simulink model "quadcopter_wind"  (Simulink 9.0)
settings: Solver=ode45  StartTime=0.0  StopTime=30  FixedStep=0.001  RelTol=1e-3  EnableMultiTasking=on
values from neighbouring files (symbols this model uses):
  C = 1    [control_params.m]
  f_phi = 10    [control_params.m]
  f_psi = 0.1    [control_params.m]
  f_theta = 0.1    [control_params.m]
  f_x = 10    [control_params.m]
  f_y = 10    [control_params.m]
  f_z = 10    [control_params.m]
  g = 9.8    [control_params.m]
  J_1 = 1    [control_params.m]
  J_2 = 1    [control_params.m]
  J_3 = 1    [control_params.m]
  l = 0.5    [control_params.m]
  m = 1    [control_params.m]
  mu_1 = 10    [control_params.m]
  mu_2 = 2    [control_params.m]
  mu_3 = 2    [control_params.m]
  mu_4 = 10    [control_params.m]
  mu_5 = 10    [control_params.m]
  mu_6 = 10    [control_params.m]
  phi_desired = 20    [control_params.m]
  sigma_1 = 30    [control_params.m]
  sigma_2 = 30    [control_params.m]
  sigma_3 = 30    [control_params.m]
  sigma_4 = 30    [control_params.m]
  sigma_5 = 30    [control_params.m]
  sigma_6 = 30    [control_params.m]
  x_desired = 10    [control_params.m]
  y_desired = 20    [control_params.m]
  z_desired = 30    [control_params.m]
settings Model: Creator=Oleg Borisov  LastModifiedBy=broth
settings DataIOCC: LimitDataPoints=on  SignalLoggingSaveFormat=ModelDataLogs
settings OptimizationCC: ExpressionDepthLimit=2147483647
settings DebuggingCC: SolverPrmCheckMsg=warning  FcnCallInpInsideContextMsg=warning  StateNameClashWarn=warning
settings GRTTargetCC: GeneratePreprocessorConditionals=Disable all  CombineOutputUpdateFcns=off  GRTInterface=on

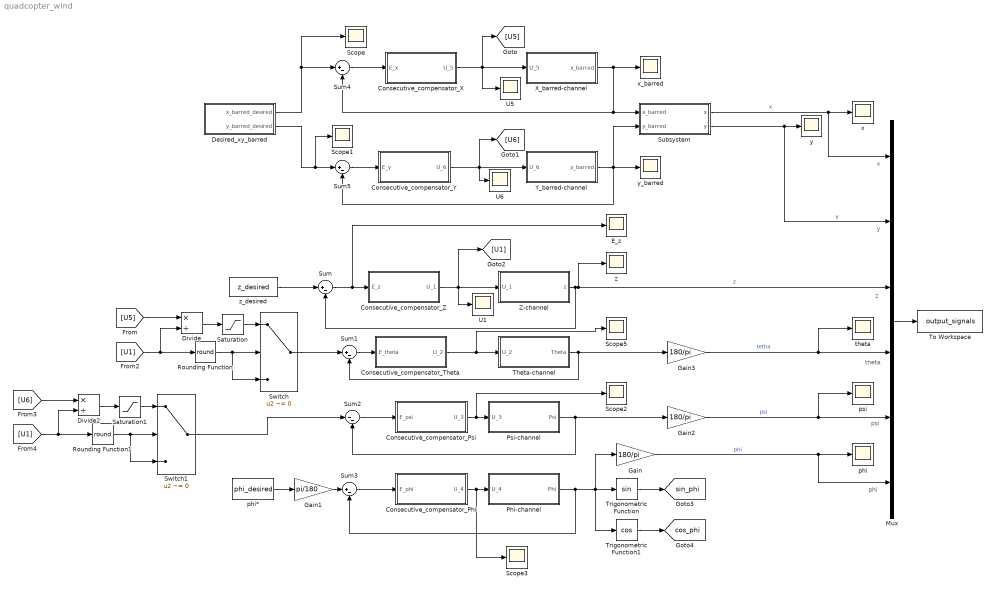
== system quadcopter_wind ==
  note: z
  note: y
  note: x
  note: theta
  note: psi
  note: phi
  Consecutive_compensator_Phi : Subsystem
  Consecutive_compensator_Psi : Subsystem
  Consecutive_compensator_Theta : Subsystem
  Consecutive_compensator_X : Subsystem
  Consecutive_compensator_Y : Subsystem
  Consecutive_compensator_Z : Subsystem
  Desired_xy_barred : Subsystem
  Divide : Product  Inputs=*/
  Divide2 : Product  Inputs=*/
  E_z : Scope
  Gain : Gain  Gain=180/pi
  Gain1 : Gain  Gain=pi/180
  Gain2 : Gain  Gain=180/pi
  Gain3 : Gain  Gain=180/pi
  Mux : Mux  Inputs=6
  Phi-channel : Subsystem
  Psi-channel : Subsystem
  Rounding Function : Rounding  Operator=round
  Rounding Function1 : Rounding  Operator=round
  Saturation : Saturate  UpperLimit=pi/6  LowerLimit=-pi/6
  Saturation1 : Saturate  UpperLimit=pi/6  LowerLimit=-pi/6
  Scope{,1..3,5} (5 alike) : Scope
  Subsystem : Subsystem
  Sum{,1,3..5} (5 alike) : Sum  Inputs=|+-
  Sum2 : Sum  Inputs=|--
  Switch : Switch  Criteria=u2 ~= 0
  Switch1 : Switch  Criteria=u2 ~= 0
  Theta-channel : Subsystem
  To Workspace : ToWorkspace  VariableName=output_signals  SaveFormat=Structure With Time  SampleTime=-1
  Trigonometric Function : Trigonometry
  Trigonometric Function1 : Trigonometry  Operator=cos
  U1 : Scope
  U5 : Scope
  U6 : Scope
  X_barred-channel : Subsystem
  Y_barred-channel : Subsystem
  Z-channel : Subsystem
  phi : Scope
  phi* : Constant  Value=phi_desired
  psi : Scope
  theta : Scope
  x : Scope
  x_barred : Scope
  y : Scope
  y_barred : Scope
  z : Scope
  z_desired : Constant  Value=z_desired
  tag scope: cos_phi=global, sin_phi=global
  wires:
  Z-channel/1(z) -> Mux/3, z/1, Sum/2  "z"
  Sum/1 -> E_z/1, Consecutive_compensator_Z/1(E_z)
  Consecutive_compensator_Psi/1(U_3) -> Psi-channel/1(U_3), Scope2/1
  Consecutive_compensator_Phi/1(U_4) -> Phi-channel/1(U_4), Scope3/1
  Theta-channel/1(Theta) -> Sum1/2, Gain3/1
  Sum1/1 -> Consecutive_compensator_Theta/1(E_theta)
  Sum2/1 -> Consecutive_compensator_Psi/1(E_psi)
  Psi-channel/1(Psi) -> Sum2/2, Gain2/1
  Sum3/1 -> Consecutive_compensator_Phi/1(E_phi)
  Phi-channel/1(Phi) -> Sum3/2, Trigonometric Function/1, Trigonometric Function1/1, Gain/1
  Consecutive_compensator_Y/1(U_6) -> Y_barred-channel/1(U_6), [U6], U6/1
  [U5] -> Divide/1
  X_barred-channel/1(x_barred) -> x_barred/1, Subsystem/1(x_barred), Sum4/2
  Sum5/1 -> Consecutive_compensator_Y/1(E_y)
  Y_barred-channel/1(y_barred) -> y_barred/1, Sum5/2, Subsystem/2(y_barred)
  Desired_xy_barred/1(x_barred_desired) -> Sum4/1, Scope/1
  Desired_xy_barred/2(y_barred_desired) -> Sum5/1, Scope1/1
  Trigonometric Function/1 -> [sin_phi]
  Trigonometric Function1/1 -> [cos_phi]
  Gain/1 -> Mux/6, phi/1  "phi"
  phi*/1 -> Gain1/1
  Gain1/1 -> Sum3/1
  Mux/1 -> To Workspace/1
  Subsystem/1(x) -> Mux/1, x/1  "x"
  Subsystem/2(y) -> Mux/2, y/1  "y"
  Gain2/1 -> Mux/5, psi/1  "psi"
  Gain3/1 -> Mux/4, theta/1  "tetha"
  Sum4/1 -> Consecutive_compensator_X/1(E_x)
  Consecutive_compensator_X/1(U_5) -> X_barred-channel/1(U_5), [U5], U5/1
  Consecutive_compensator_Z/1(U_1) -> Z-channel/1(U_1), [U1], U1/1
  z_desired/1 -> Sum/1
  Divide/1 -> Saturation/1
  [U1] -> Divide/2, Rounding Function/1
  Switch/1 -> Sum1/1
  Saturation/1 -> Switch/1
  Rounding Function/1 -> Switch/2, Switch/3
  Consecutive_compensator_Theta/1(U_2) -> Theta-channel/1(U_2), Scope5/1
  [U6] -> Divide2/1
  Divide2/1 -> Saturation1/1
  [U1] -> Divide2/2, Rounding Function1/1
  Saturation1/1 -> Switch1/1
  Rounding Function1/1 -> Switch1/2, Switch1/3
  Switch1/1 -> Sum2/1

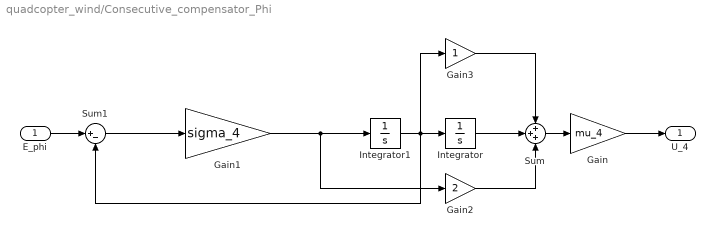
== system quadcopter_wind/Consecutive_compensator_Phi ==
  E_phi : Inport
  Gain : Gain  Gain=mu_4
  Gain1 : Gain  Gain=sigma_4
  Gain2 : Gain  Gain=2
  Gain3 : Gain
  Integrator : Integrator
  Integrator1 : Integrator
  Sum : Sum  Inputs=+++
  Sum1 : Sum  Inputs=|+-
  U_4 : Outport
  wires:
  Sum/1 -> Gain/1
  Integrator/1 -> Sum/2
  Sum1/1 -> Gain1/1
  Gain/1 -> U_4/1
  Integrator1/1 -> Integrator/1, Gain3/1, Sum1/2
  Gain1/1 -> Integrator1/1, Gain2/1
  Gain3/1 -> Sum/1
  E_phi/1 -> Sum1/1
  Gain2/1 -> Sum/3

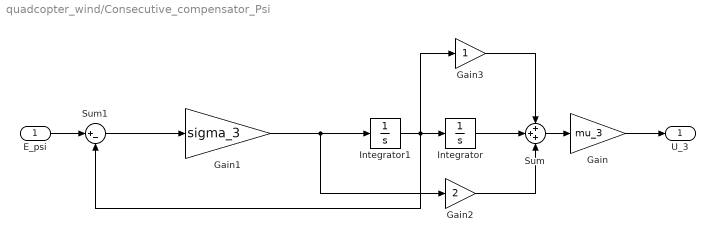
== system quadcopter_wind/Consecutive_compensator_Psi ==
  E_psi : Inport
  Gain : Gain  Gain=mu_3
  Gain1 : Gain  Gain=sigma_3
  Gain2 : Gain  Gain=2
  Gain3 : Gain
  Integrator : Integrator
  Integrator1 : Integrator
  Sum : Sum  Inputs=+++
  Sum1 : Sum  Inputs=|+-
  U_3 : Outport
  wires:
  Sum/1 -> Gain/1
  Sum1/1 -> Gain1/1
  Gain/1 -> U_3/1
  Integrator1/1 -> Integrator/1, Gain3/1, Sum1/2
  Gain1/1 -> Integrator1/1, Gain2/1
  Gain3/1 -> Sum/1
  E_psi/1 -> Sum1/1
  Integrator/1 -> Sum/2
  Gain2/1 -> Sum/3

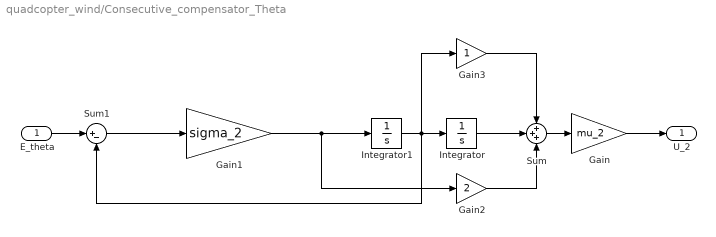
== system quadcopter_wind/Consecutive_compensator_Theta ==
  E_theta : Inport
  Gain : Gain  Gain=mu_2
  Gain1 : Gain  Gain=sigma_2
  Gain2 : Gain  Gain=2
  Gain3 : Gain
  Integrator : Integrator
  Integrator1 : Integrator
  Sum : Sum  Inputs=+++
  Sum1 : Sum  Inputs=|+-
  U_2 : Outport
  wires:
  Sum/1 -> Gain/1
  Sum1/1 -> Gain1/1
  Gain/1 -> U_2/1
  Integrator1/1 -> Integrator/1, Gain3/1, Sum1/2
  Gain1/1 -> Integrator1/1, Gain2/1
  Gain3/1 -> Sum/1
  E_theta/1 -> Sum1/1
  Integrator/1 -> Sum/2
  Gain2/1 -> Sum/3

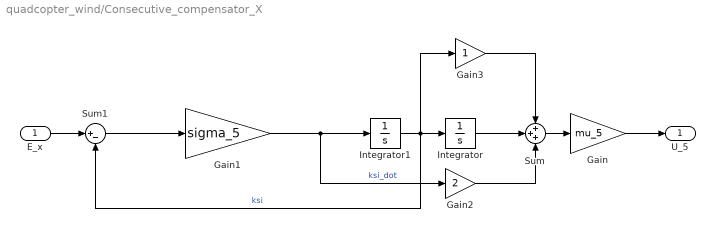
== system quadcopter_wind/Consecutive_compensator_X ==
  E_x : Inport
  Gain : Gain  Gain=mu_5
  Gain1 : Gain  Gain=sigma_5
  Gain2 : Gain  Gain=2
  Gain3 : Gain
  Integrator : Integrator
  Integrator1 : Integrator
  Sum : Sum  Inputs=+++
  Sum1 : Sum  Inputs=|+-
  U_5 : Outport
  wires:
  Sum/1 -> Gain/1
  Integrator/1 -> Sum/2
  Sum1/1 -> Gain1/1
  Gain/1 -> U_5/1
  Integrator1/1 -> Integrator/1, Gain3/1, Sum1/2  "ksi"
  Gain1/1 -> Integrator1/1, Gain2/1  "ksi_dot"
  Gain3/1 -> Sum/1
  E_x/1 -> Sum1/1
  Gain2/1 -> Sum/3

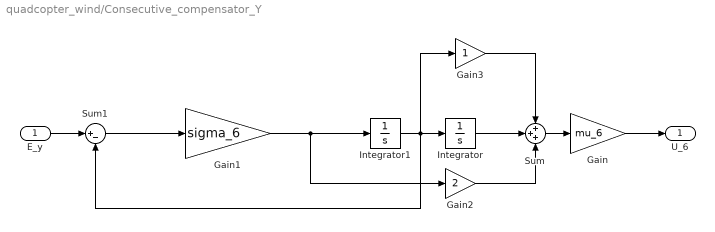
== system quadcopter_wind/Consecutive_compensator_Y ==
  E_y : Inport
  Gain : Gain  Gain=mu_6
  Gain1 : Gain  Gain=sigma_6
  Gain2 : Gain  Gain=2
  Gain3 : Gain
  Integrator : Integrator
  Integrator1 : Integrator
  Sum : Sum  Inputs=+++
  Sum1 : Sum  Inputs=|+-
  U_6 : Outport
  wires:
  Sum/1 -> Gain/1
  Integrator/1 -> Sum/2
  Sum1/1 -> Gain1/1
  Gain/1 -> U_6/1
  Integrator1/1 -> Integrator/1, Gain3/1, Sum1/2
  Gain1/1 -> Integrator1/1, Gain2/1
  Gain3/1 -> Sum/1
  E_y/1 -> Sum1/1
  Gain2/1 -> Sum/3

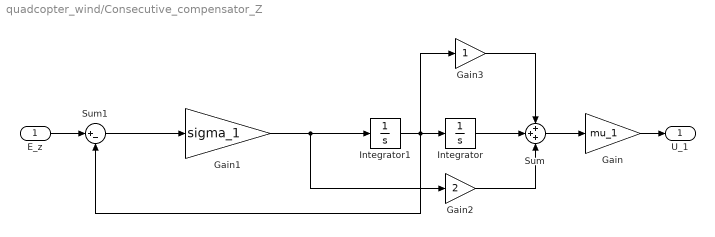
== system quadcopter_wind/Consecutive_compensator_Z ==
  E_z : Inport
  Gain : Gain  Gain=mu_1
  Gain1 : Gain  Gain=sigma_1
  Gain2 : Gain  Gain=2
  Gain3 : Gain
  Integrator : Integrator
  Integrator1 : Integrator
  Sum : Sum  Inputs=+++
  Sum1 : Sum  Inputs=|+-
  U_1 : Outport
  wires:
  Sum/1 -> Gain/1
  Integrator/1 -> Sum/2
  Sum1/1 -> Gain1/1
  Integrator1/1 -> Integrator/1, Gain3/1, Sum1/2
  Gain1/1 -> Integrator1/1, Gain2/1
  Gain3/1 -> Sum/1
  Gain/1 -> U_1/1
  E_z/1 -> Sum1/1
  Gain2/1 -> Sum/3

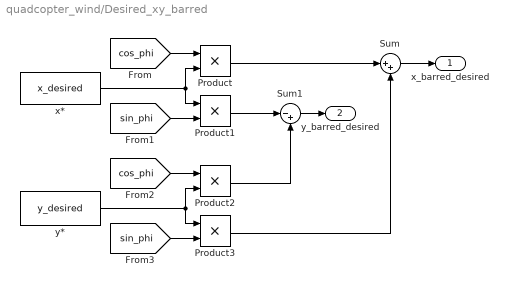
== system quadcopter_wind/Desired_xy_barred ==
  Product{,1..3} (4 alike) : Product  RndMeth=Zero
  Sum : Sum  Inputs=|++
  Sum1 : Sum  Inputs=|-+
  x* : Constant  Value=x_desired
  y* : Constant  Value=y_desired
  x_barred_desired : Outport
  y_barred_desired : Outport  Port=2
  wires:
  [cos_phi] -> Product/1
  [sin_phi] -> Product1/2
  [cos_phi] -> Product2/1
  [sin_phi] -> Product3/2
  Product/1 -> Sum/1
  Product3/1 -> Sum/2
  Product1/1 -> Sum1/1
  Product2/1 -> Sum1/2
  Sum/1 -> x_barred_desired/1
  Sum1/1 -> y_barred_desired/1
  x*/1 -> Product/2, Product1/1
  y*/1 -> Product2/2, Product3/1

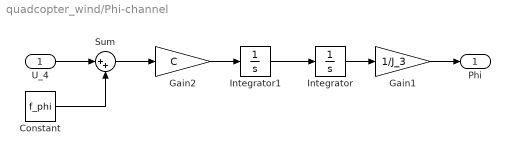
== system quadcopter_wind/Phi-channel ==
  U_4 : Inport
  Constant : Constant  Value=f_phi
  Gain1 : Gain  Gain=1/J_3
  Gain2 : Gain  Gain=C
  Integrator : Integrator
  Integrator1 : Integrator
  Sum : Sum  Inputs=|++
  Phi : Outport
  wires:
  Integrator1/1 -> Integrator/1
  Integrator/1 -> Gain1/1
  Gain1/1 -> Phi/1
  Gain2/1 -> Integrator1/1
  U_4/1 -> Sum/1
  Sum/1 -> Gain2/1
  Constant/1 -> Sum/2

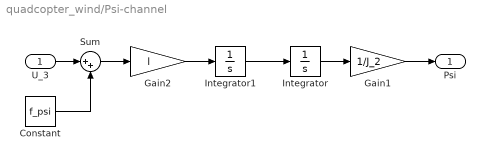
== system quadcopter_wind/Psi-channel ==
  U_3 : Inport
  Constant : Constant  Value=f_psi
  Gain1 : Gain  Gain=1/J_2
  Gain2 : Gain  Gain=l
  Integrator : Integrator
  Integrator1 : Integrator
  Sum : Sum  Inputs=|++
  Psi : Outport
  wires:
  Integrator1/1 -> Integrator/1
  Integrator/1 -> Gain1/1
  Gain1/1 -> Psi/1
  Gain2/1 -> Integrator1/1
  U_3/1 -> Sum/1
  Sum/1 -> Gain2/1
  Constant/1 -> Sum/2

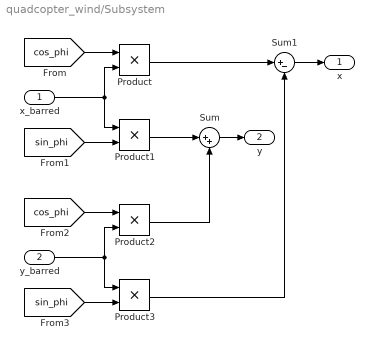
== system quadcopter_wind/Subsystem ==
  x_barred : Inport
  y_barred : Inport  Port=2
  Product{,1..3} (4 alike) : Product  RndMeth=Zero
  Sum : Sum  Inputs=|++
  Sum1 : Sum  Inputs=|+-
  x : Outport
  y : Outport  Port=2
  wires:
  [cos_phi] -> Product/1
  [sin_phi] -> Product1/2
  x_barred/1 -> Product/2, Product1/1
  [cos_phi] -> Product2/1
  [sin_phi] -> Product3/2
  y_barred/1 -> Product2/2, Product3/1
  Product1/1 -> Sum/1
  Product2/1 -> Sum/2
  Product/1 -> Sum1/1
  Product3/1 -> Sum1/2
  Sum1/1 -> x/1
  Sum/1 -> y/1

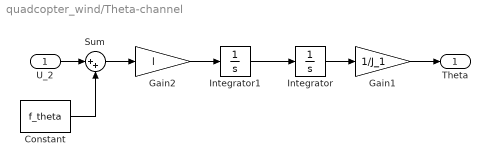
== system quadcopter_wind/Theta-channel ==
  U_2 : Inport
  Constant : Constant  Value=f_theta
  Gain1 : Gain  Gain=1/J_1
  Gain2 : Gain  Gain=l
  Integrator : Integrator
  Integrator1 : Integrator
  Sum : Sum  Inputs=|++
  Theta : Outport
  wires:
  Integrator1/1 -> Integrator/1
  Integrator/1 -> Gain1/1
  Gain1/1 -> Theta/1
  Gain2/1 -> Integrator1/1
  U_2/1 -> Sum/1
  Sum/1 -> Gain2/1
  Constant/1 -> Sum/2

== system quadcopter_wind/X_barred-channel ==
  U_5 : Inport
  Constant : Constant  Value=f_x
  Gain1 : Gain  Gain=1/m
  Integrator : Integrator
  Integrator1 : Integrator
  Sum : Sum  Inputs=|++
  x_barred : Outport
  wires:
  Integrator1/1 -> Integrator/1
  Integrator/1 -> Gain1/1
  Gain1/1 -> x_barred/1
  U_5/1 -> Sum/1
  Sum/1 -> Integrator1/1
  Constant/1 -> Sum/2

== system quadcopter_wind/Y_barred-channel ==
  U_6 : Inport
  Constant : Constant  Value=f_y
  Gain1 : Gain  Gain=1/m
  Integrator : Integrator
  Integrator1 : Integrator
  Sum : Sum  Inputs=|++
  y_barred : Outport
  wires:
  Integrator1/1 -> Integrator/1
  Integrator/1 -> Gain1/1
  Gain1/1 -> y_barred/1
  U_6/1 -> Sum/1
  Sum/1 -> Integrator1/1
  Constant/1 -> Sum/2

== system quadcopter_wind/Z-channel ==
  U_1 : Inport
  Constant : Constant  Value=m*g
  Constant1 : Constant  Value=f_z
  Gain1 : Gain  Gain=1/m
  Integrator : Integrator
  Integrator1 : Integrator
  Sum : Sum  Inputs=++-
  z : Outport
  wires:
  Sum/1 -> Integrator1/1
  Integrator1/1 -> Integrator/1
  Integrator/1 -> Gain1/1
  Gain1/1 -> z/1
  Constant/1 -> Sum/3
  U_1/1 -> Sum/2
  Constant1/1 -> Sum/1
